simulink model "estimation_data_with_new_parameter_new"  (R2022a)
settings: Solver=VariableStepDiscrete  StartTime=0.0  StopTime=inf  FixedStep=0.1  RelTol=1e-8
values from neighbouring files (symbols this model uses):
  L3 = Y*inv(P)    [lqr_synthesis_observer_simple_Lx3x3_no_VOC.m]
libraries: simulink x1, eeDiscretePi x1
settings Model: Creator=spinolam  LastModifiedBy=spinolam

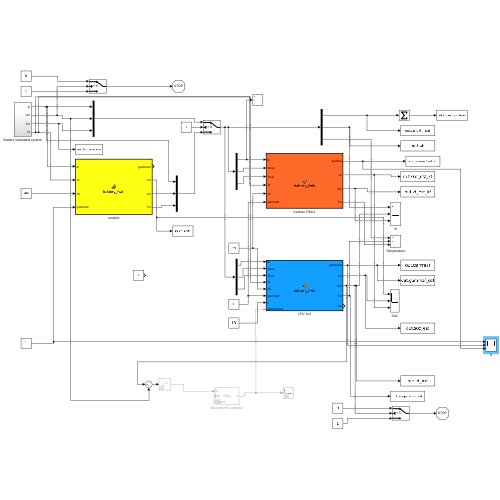
[thumbnail: Simulink's stored preview of the top-level diagram]
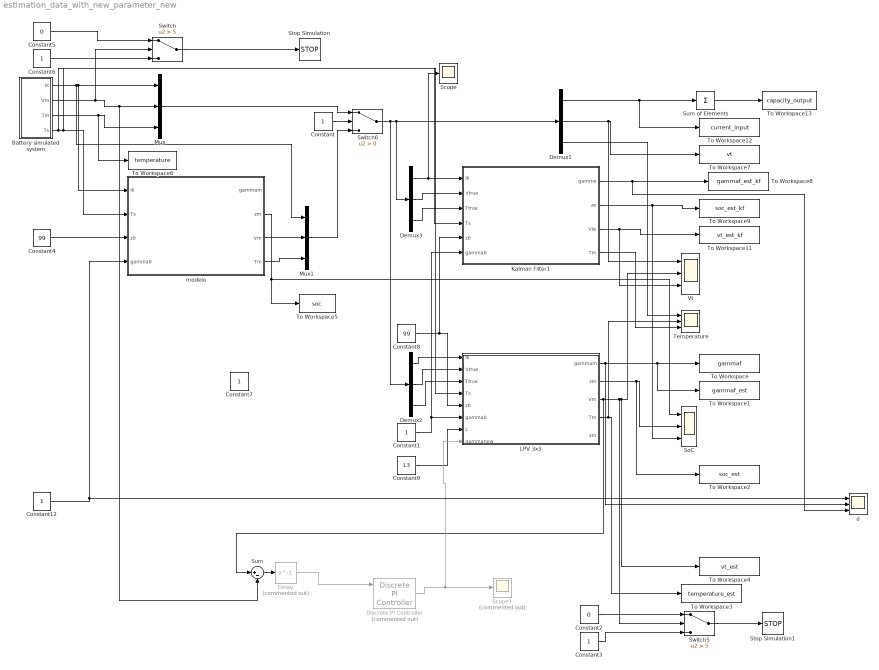
== system estimation_data_with_new_parameter_new ==
  Battery simulated system : Subsystem
  Constant : Constant
  Constant1 : Constant  SampleTime=-1
  Constant12 : Constant  SampleTime=-1
  Constant2 : Constant  Value=0
  Constant3 : Constant
  Constant4 : Constant  Value=99  SampleTime=-1
  Constant5 : Constant  Value=0
  Constant6 : Constant
  Constant7 : Constant  SampleTime=-1
  Constant8 : Constant  Value=99  SampleTime=-1
  Constant9 : Constant  Value=L3  SampleTime=-1
  Delay : Delay  Commented=on  DelayLength=1
  Demux1 : Demux  Outputs=3
  Demux2 : Demux  Outputs=3
  Demux3 : Demux  Outputs=3
  Discrete PI Controller : eeDiscretePi/Discrete PI Controller  Commented=on  Kp=0.1  Ki=0.1  Kaw=1  x0=1  Ts=1
      settings: SourceProductBaseCode=PS
  Kalman Filter1 : MATLAB Function  TreatAsAtomicUnit=on
  LPV 3x3 : MATLAB Function  TreatAsAtomicUnit=on  SystemSampleTime=1
  Mux : Mux  Inputs=3
  Mux1 : Mux  Inputs=3
  Scope : Scope
  Scope1 : Scope  Commented=on
  SoC : Scope  NumInputPorts=3
  Stop Simulation : Stop
  Stop Simulation1 : Stop
  Sum : Sum  Inputs=|+-
  Sum of Elements : Sum  Inputs=+
  Switch : Switch  Criteria=u2 > Threshold  Threshold=5  SaturateOnIntegerOverflow=off  InputSameDT=off
  Switch5 : Switch  Criteria=u2 > Threshold  Threshold=5  SaturateOnIntegerOverflow=off  InputSameDT=off
  Switch6 : Switch  Criteria=u2 > Threshold  SaturateOnIntegerOverflow=off  InputSameDT=off
  Temperature : Scope  NumInputPorts=3
  To Workspace : ToWorkspace  VariableName=gammaf  SampleTime=-1
  To Workspace1 : ToWorkspace  VariableName=gammaf_est  SampleTime=-1
  To Workspace11 : ToWorkspace  VariableName=vt_est_kf  SampleTime=-1
  To Workspace12 : ToWorkspace  VariableName=current_input  SampleTime=-1
  To Workspace13 : ToWorkspace  VariableName=capacity_output  SampleTime=-1
  To Workspace2 : ToWorkspace  VariableName=soc_est  SampleTime=-1
  To Workspace3 : ToWorkspace  VariableName=temperature_est  SampleTime=-1
  To Workspace4 : ToWorkspace  VariableName=vt_est  SampleTime=-1
  To Workspace5 : ToWorkspace  VariableName=soc  SampleTime=-1
  To Workspace6 : ToWorkspace  VariableName=temperature  SampleTime=-1
  To Workspace7 : ToWorkspace  VariableName=vt  SampleTime=-1
  To Workspace8 : ToWorkspace  VariableName=gammaf_est_kf  SampleTime=-1
  To Workspace9 : ToWorkspace  VariableName=soc_est_kf  SampleTime=-1
  Vt : Scope  NumInputPorts=3
  d : Scope  NumInputPorts=3
  modelo : MATLAB Function  TreatAsAtomicUnit=on
  wires:
  LPV 3x3/2(zm) -> To Workspace2/1, SoC/2
  LPV 3x3/3(Vm) -> To Workspace4/1, Vt/2, Switch5/2, Sum/1
  Kalman Filter1/1(gamme) -> d/3, To Workspace8/1
  Kalman Filter1/2(ze) -> SoC/3, To Workspace9/1
  Kalman Filter1/3(Vte) -> Vt/3, To Workspace11/1
  Battery simulated system/1(Ik) -> modelo/1(Ik), Mux/1, Mux1/1
  Switch/1 -> Stop Simulation/1
  Demux2/1 -> LPV 3x3/1(Ik)
  modelo/2(zm) -> SoC/1, To Workspace5/1
  Constant5/1 -> Switch/1
  Demux2/2 -> LPV 3x3/2(Vtrue)
  Constant3/1 -> Switch5/3
  Mux/1 -> Switch6/1
  Constant8/1 -> Kalman Filter1/5(z0), LPV 3x3/5(z0)
  Kalman Filter1/4(Tm) -> Temperature/3
  Demux1/2 -> Vt/1, To Workspace7/1
  Demux3/2 -> Kalman Filter1/2(Vtrue)
  Demux3/3 -> Kalman Filter1/3(Ttrue)
  LPV 3x3/4(Tm) -> To Workspace3/1, Temperature/2
  Switch5/1 -> Stop Simulation1/1
  Mux1/1 -> Switch6/3
  Sum of Elements/1 -> To Workspace13/1
  Constant4/1 -> modelo/3(z0)
  Constant/1 -> Switch6/2
  Battery simulated system/3(Tm) -> To Workspace6/1, Mux/3
  Demux1/1 -> Sum of Elements/1, To Workspace12/1
  Demux1/3 -> Temperature/1
  Demux3/1 -> Scope/1, Kalman Filter1/1(Ik)
  Constant9/1 -> LPV 3x3/7(L)
  Constant2/1 -> Switch5/1
  Constant6/1 -> Switch/3
  modelo/4(Tm) -> Mux1/3
  modelo/3(Vm) -> Mux1/2
  Demux2/3 -> LPV 3x3/3(Ttrue)
  Battery simulated system/4(Ts) -> LPV 3x3/4(Ts), Kalman Filter1/4(Ts), modelo/2(Ts)
  Constant1/1 -> LPV 3x3/6(gamma0), Kalman Filter1/6(gamma0)
  Switch6/1 -> Demux3/1, Demux1/1, Demux2/1
  Sum/1 -> Delay/1
  Battery simulated system/2(Vm) -> Switch/2, Sum/2, Mux/2
  Discrete PI Controller/1 -> LPV 3x3/8(gammanew), Scope1/1
  Delay/1 -> Discrete PI Controller/1
  LPV 3x3/1(gammam) -> d/2, To Workspace1/1, To Workspace/1
  Constant12/1 -> d/1, modelo/4(gamma0)

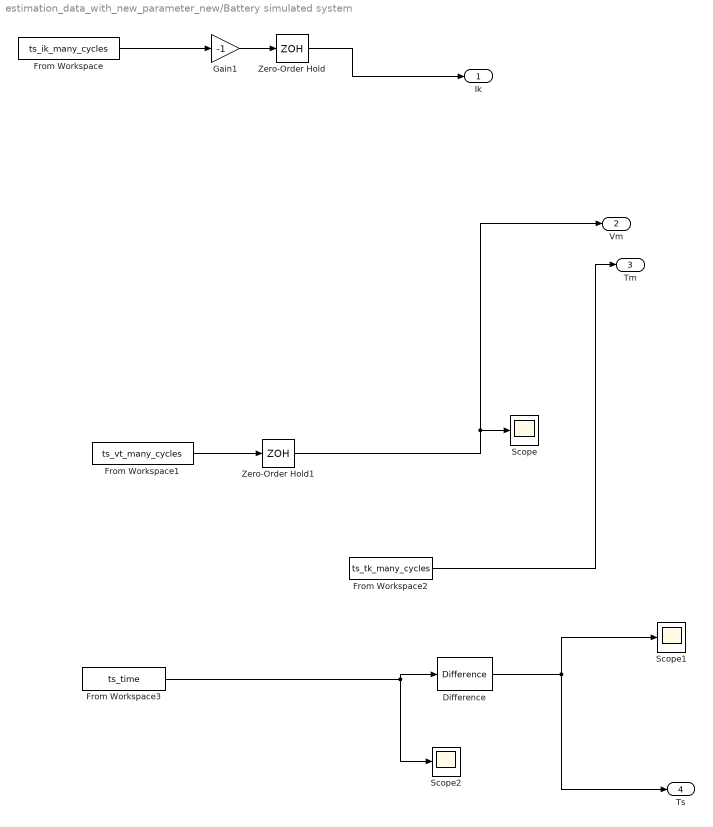
== system estimation_data_with_new_parameter_new/Battery simulated system ==
  Difference : simulink/Discrete/Difference  ICPrevInput=0.0  OutMin=[]  OutMax=[]  OutDataType=fixdt(1, 16)  OutScaling=2^-10  DoSatur=off
  From Workspace : FromWorkspace  VariableName=ts_ik_many_cycles  SampleTime=1  Interpolate=off  ZeroCross=off  OutputAfterFinalValue=Setting to zero
  From Workspace1 : FromWorkspace  VariableName=ts_vt_many_cycles  SampleTime=1  Interpolate=off  ZeroCross=off  OutputAfterFinalValue=Setting to zero
  From Workspace2 : FromWorkspace  VariableName=ts_tk_many_cycles  SampleTime=1  Interpolate=off  ZeroCross=off  OutputAfterFinalValue=Setting to zero
  From Workspace3 : FromWorkspace  VariableName=ts_time  OutDataTypeStr=double  SampleTime=1  Interpolate=off  ZeroCross=off  OutputAfterFinalValue=Setting to zero
  Gain1 : Gain  Gain=-1
  Scope : Scope
  Scope1 : Scope
  Scope2 : Scope
  Zero-Order Hold : ZeroOrderHold  SampleTime=-1
  Zero-Order Hold1 : ZeroOrderHold  SampleTime=-1
  Ik : Outport
  Vm : Outport  Port=2
  Tm : Outport  Port=3
  Ts : Outport  Port=4
  wires:
  From Workspace2/1 -> Tm/1
  From Workspace/1 -> Gain1/1
  From Workspace3/1 -> Difference/1, Scope2/1
  Difference/1 -> Scope1/1, Ts/1
  From Workspace1/1 -> Zero-Order Hold1/1
  Gain1/1 -> Zero-Order Hold/1
  Zero-Order Hold/1 -> Ik/1
  Zero-Order Hold1/1 -> Vm/1, Scope/1

== matlab function estimation_data_with_new_parameter_new/LPV 3x3 ==
  data: Ik input; Vtrue input; Ttrue input; Ts input; gammam output; zm output; Vm output; Tm output; z0 input; gamma0 input; L input; xm output; gammanew input
function [gammam,zm,Vm, Tm,xm]= battery_twin(Ik,Vtrue,Ttrue,Ts, z0, gamma0,L,gammanew)

persistent zk Vk Tk gammak x Tamb

% params_opt =[0.610556521150227
%    8.598775712524340
%    0.122603898484246
%    2.606767267852760
%    0.192039393270390
%   -0.001348398288203
%    0.000025296007798
%   -0.000000662621556
%    0.000000004414584
%    0.996817945207983
%    2.298831860870833
%   23.000000000000000
% 
% 
% ];
params_opt =[0.919813763352173
   8.599767631518853
   0.273094682411476
   5.142135137038677
   0.094988476730227
  -0.002370241318109
   0.000090365520095
  -0.000001529036050
   0.000000008558929
   0.999025068018285
   8.420763231826188
  23.336063234459374
];
params_opt=[0.919813763352173
   8.599767631518853
   0.273094682411476
   5.142135137038677
   0.094988476730227
  -0.002370241318109
   0.000090365520095
  -0.000001529036050
   0.000000008558929
   0.999025068018285
   8.420763231826188
  23.336063234459374];

params_opt=[0.589068193185747
   8.559272902690564
   0.048189025436034
   3.256250824353102
   0.217261878522855
  -0.000962410714053
   0.000009822495048
  -0.000000423528870
   0.000000002938409
   0.994927725009115
   1.937154456656148
  23.000000000000000];

% --- Parameters Battery ---
N=1;

a=params_opt(1);
% Parameters model Voc
Eo=params_opt(2);
K1=params_opt(3);
K2=params_opt(4);


R0=params_opt(5);
R1=params_opt(6);
R2=params_opt(7);
R3=params_opt(8);
R4=params_opt(9);


%Nominal capacity
Cr =2.5;

% Parameters model temperature
%c2 = 4;
b=params_opt(10); 
c1=params_opt(11);
%Tamb = params_opt(12);
% % --- Parameters Battery ---
% N=1;
% b=0.999; 
% a=0.724851923449880;
% % Parameters model Voc
% Eo=8.455947458036864;
% K1=0.144592227425476;
% K2=0.607377452866854;
% 
% 
% R0=0.216916476498134;
% R1=-0.005249797087054;
% R2=0.000141179901879;
% R3=-0.000002104480344;
% R4=0.000000010785500;
% 
% 
% %Nominal capacity
% Cr =2.5;
% 
% % Parameters model temperature
% %c2 = 4;
% c1=4;
% %Tamb = 23;

% -- Values LPV
%L=[-0.7386   14.3891    0.4483];

%L=0*[-0.270468799102130 0.551733258663858 0.289617027889015];
% N=1;
% b=0.997542721848054; 
% a=0.724851923449880;
% % Parameters model Voc
% Eo=8.455947458036864;
% K1=0.144592227425476;
% K2=0.607377452866854;
% 
% 
% R0=0.216916476498134;
% R1=-0.005249797087054;
% R2=0.000141179901879;
% R3=-0.000002104480344;
% R4=0.000000010785500;
% 
% 
% %Nominal capacity
% Cr =2.5;
% 
% % Parameters model temperature
% %c2 = 4;
% c1=2.310386631071339;
% --- initial states ----
Ik=-Ik;
if isempty(gammak)
    gammak=gamma0;
    
end
if isempty(zk)
    zk=z0;
end
if isempty(Vk) 
    Vk=N*Eo; 
end
if isempty(Tk)
    Tamb=Ttrue; 
    Tk=Tamb; 
end
if isempty(x)
    x=[gamma0;z0;Eo];
end

%L=0*L;
if zk>99.9
    zk=99.9;
end
if zk>99.9
    zk=99.9;
end

% --- map functions -----
Rint=(R0+R1*zk+R2*zk^2+R3*zk^3+R4*zk^4);
Voc=(Eo-K1*log(100-zk)-K2/zk);

% --- dynamic model -----
error=(Vtrue-Vk);
%L=[-0.279587147260702
 %  1.066424440638722
  % 0.267404777088713]';
% --- dynamic model -----
rho1= -100*Ik/(3600*Cr)*Ts;
Rint=N*(R0+R1*x(2)+R2*x(2)^2+R3*x(2)^3+R4*x(2)^4);
rho2= -Ik*Rint;
%Voc=N*(Eo-K1*log(100-x(2))-K2/x(2));
%rho3= Voc/x(2);

L=L;
gamma1 =  1*gammak + L(1)*error;


z1 = zk - Ts*Ik*100*gammak/(3600*Cr)+ L(2)*error;


Ek = Voc-(Rint)*Ik*gammak;
V1 = a*Vk + (1-a)*Ek + L(3)*error;

Tj= Rint*gammak*Ik^2;
T1 = b*Tk + (1-b)*(c1*Tj+Tamb);

A =[ 1 0 0 
       rho1 1 0 
       (1-a)*rho2 0 a ];

B=[0 0 (1-a)*Voc]';
x1 = A*x + B*1+ L*error;

    %sensor model:
zm = zk; % + noise
Vm = Vk; % + noise
gammam =gammak;
Tm=Tk;
xm=x;
%updating z:
x=x1;
zk = z1;
Vk = V1;
Tk=T1;
gammak=gamma1;

== matlab function estimation_data_with_new_parameter_new/modelo ==
  data: Ik input; Ts input; gammam output; zm output; Vm output; Tm output; z0 input; gamma0 input
function [gammam,zm,Vm, Tm]= battery_twin(Ik,Ts, z0, gamma0)

persistent zk Vk Tk gammak

% --- Parameters Battery ---
N=1;
b=0.997542721848054; 
a=0.724851923449880;
% Parameters model Voc
Eo=8.455947458036864;
K1=0.144592227425476;
K2=0.607377452866854;


R0=0.216916476498134;
R1=-0.005249797087054;
R2=0.000141179901879;
R3=-0.000002104480344;
R4=0.000000010785500;


%Nominal capacity
Cr =2.5;

% Parameters model temperature
%c2 = 4;
c1=2.310386631071339;
Tamb = 23;

% -- Values LPV
%L=[-0.7386   14.3891    0.4483];

%L=0*[-0.270468799102130 0.551733258663858 0.289617027889015];
% --- initial states ----
Ik=-Ik;
if isempty(gammak)
    gammak=gamma0;
end
if isempty(zk)
    zk=z0;
end
if isempty(Vk) 
    Vk=N*Eo; 
end
if isempty(Tk)
    Tk=Tamb; 
end

if zk>99.9
    zk=99.9;
end

% --- map functions -----
Rint=(R0+R1*zk+R2*zk^2+R3*zk^3+R4*zk^4);
Voc=(Eo-K1*log(100-zk)-K2/zk);

% --- dynamic model -----




gamma1 =  1*gammak ;

z1 = zk - Ts*Ik*100*gammak/(3600*Cr);


Ek = Voc-(Rint)*Ik*gammak;
V1 = a*Vk + (1-a)*Ek;


Tj= Rint*gammak*Ik^2;
T1 = b*Tk + (1-b)*(c1*Tj+Tamb);

    %sensor model:
zm = zk; % + noise
Vm = Vk; % + noise
gammam =gammak;
Tm=Tk;
%updating z:

zk = z1;
Vk = V1;
Tk=T1;
gammak=gamma1;

== matlab function estimation_data_with_new_parameter_new/Kalman Filter1 ==
  data: Ik input; Vtrue input; Ttrue input; Ts input; gamme output; ze output; Vte output; z0 input; gamma0 input; Tm output
function [gamme,ze,Vte,Tm]= battery_twin(Ik,Vtrue,Ttrue,Ts ...
    , z0, gamma0)

persistent x P Tk Tamb

% % --- Parameters Battery ---
% N=1;
% b=exp(-Ts/ 50); 
% a=exp(-Ts/20);
% % Parameters model Voc
% Eo=8.108164589440493;
% K1=0.148756441041277;
% K2=1.692232704632389;
% 
% 
% R0=0.147123759027790;
% R1=-0.002816475918113;
% R2=0.000068562265922;
% R3=-0.000001200032933;
% R4=0.000000006851701;
% 
% 
% %Nominal capacity
% Cr =2.5;
% 
% % Parameters model temperature
% %c2 = 4;
% c1=3;
% Tamb = 24;
% --- Parameters Battery ---
N=1;
b=0.997542721848054; 
a=0.724851923449880;
% Parameters model Voc
Eo=8.455947458036864;
K1=0.144592227425476;
K2=0.607377452866854;


R0=0.216916476498134;
R1=-0.005249797087054;
R2=0.000141179901879;
R3=-0.000002104480344;
R4=0.000000010785500;


%Nominal capacity
Cr =2.5;

% Parameters model temperature
%c2 = 4;
c1=2.310386631071339;
%Tamb = 23;


% --- initial states ----
if isempty(x)   
    % initial deterioration: 
    x=[gamma0;z0;Eo];
end

if isempty(Tk)
    Tamb = Ttrue;
    Tk=Tamb; 
end

if isempty(P)    
    P=[5e1 0 0 ;
        0 0 0 ;
       0 0 0 ];
    P=[33.514524222311799   0.000000003893831  29.783768130399633
   0.000000003893831   0.000000002710310  -0.000000011300228
  29.783768130399633  -0.000000011300228  29.754297006017687];
    %P=1.0e-3 *[0.219216450882279  -0.000000000002299   0.582335293134520
%  -0.000000000002299   0.000000000002341  -0.000000000072372
  % 0.582335293134520  -0.000000000072372   2.446395540241941];
end


% --- dynamic model -----
Ik=-Ik;
rho1= -100*Ik/(3600*Cr)*Ts;
Rint=N*(R0+R1*x(2)+R2*x(2)^2+R3*x(2)^3+R4*x(2)^4);
rho2= -Ik*Rint;
Voc=N*(Eo-K1*log(100-x(2))-K2/x(2));
rho3= Voc/x(2);


%%%%%%%%%%%%%%%%%%%%%%%%%%%%


Q = diag([1 0 1]);
R =10;
 
%%%%%%%%%%%%%%%%%%%%%%%%%%%%
    noise = 0*randn(1);
    y = abs(Vtrue + noise); 
    
%     A =[ 1 0 0 
%    rho1 1 0 
%    (1-a)*rho2 (1-a)*rho3 a ]
    A =[ 1 0 0 
       rho1 1 0 
       (1-a)*rho2 0 a ];

    
       
    %A = eye(4)+Ts*Ac ;  %Euler approximation 
   % %A = expm(Ac*Ts);  %Exact soluti-1on (for comparison)
    
    C=[0 0 1 ];
%     B=[0 0 0]';
    B=[0 0 (1-a)*Voc]';
    
    P = A*P*A'+Q;
    K = P*C'*inv(C*P*C'+R);
    P=(eye(3)-K*C)*P;

    error=(y - C*x);
    
    x1 = A*x + B*1+ K*error;

    if x(1)< 0, x(1)=0; end
    if x(2)< 0, x(2)=0; end
    if x(3)< 0, x(3)=0; end
    %if x(4)< 0, x(4)=0; end

    gamme = x(1); 
    ze = x(2); 
    Vte = x(3); 
    Tj= Rint*x(1)*Ik^2;
    T1 = b*Tk + (1-b)*(c1*Tj+Tamb);
    Tm=Tk;
    


    %update:
    x=x1;
    Tk=T1;

end
